simulink model "Mooventure2016_Rev5"  (Simulink 7.7)
settings: Solver=FixedStepDiscrete  StartTime=0.0  StopTime=10  RelTol=1e-3
PreLoadFcn:
  | try, eval([bdroot '_setup']); catch, eval('model_setup', ''); end
InitFcn:
  | try, eval([bdroot '_setup']); catch, eval('model_setup', ''); end
undefined symbols (not defined in the file): ECM, H1, motohawk_build_version, motohawk_trunc_name, motohawk_vardec_config_group, motohawk_vardec_path, xD
libraries: MotoHawk_lib x976, motohawk_control_primitives_lib x41, simulink x27, motohawk_annotations_lib x3
(part 14 of 16)

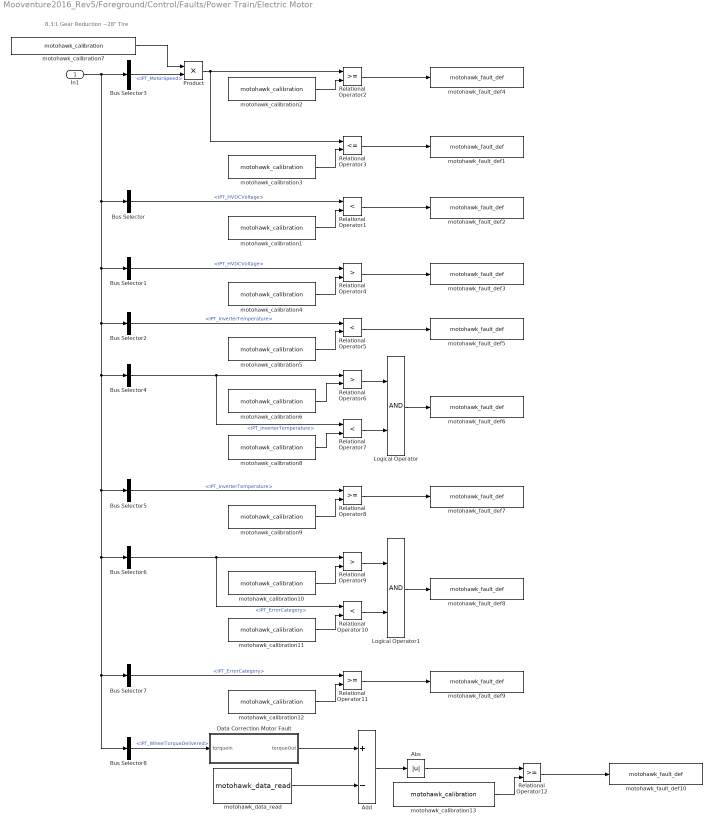
== system Mooventure2016_Rev5/Foreground/Control/Faults/Power Train/Electric Motor ==
  note: 8.3:1 Gear Reduction
      | ~28" Tire
  In1 : Inport
  Abs : Abs
  Add : Sum  Inputs=+-
  Bus Selector : BusSelector  OutputSignals=IPT.ID 278 IPT Status 1.IPT_HVDCVoltage
  Bus Selector1 : BusSelector  OutputSignals=IPT.ID 278 IPT Status 1.IPT_HVDCVoltage
  Bus Selector2 : BusSelector  OutputSignals=IPT.ID 278 IPT Status 1.IPT_InverterTemperature
  Bus Selector3 : BusSelector  OutputSignals=IPT.ID 260 IPT Status 2.IPT_MotorSpeed
  Bus Selector4 : BusSelector  OutputSignals=IPT.ID 278 IPT Status 1.IPT_InverterTemperature
  Bus Selector5 : BusSelector  OutputSignals=IPT.ID 278 IPT Status 1.IPT_InverterTemperature
  Bus Selector6 : BusSelector  OutputSignals=IPT.ID 278 IPT Status 1.IPT_ErrorCategory
  Bus Selector7 : BusSelector  OutputSignals=IPT.ID 278 IPT Status 1.IPT_ErrorCategory
  Bus Selector8 : BusSelector  OutputSignals=IPT.ID 260 IPT Status 2.IPT_WheelTorqueDelivered
  Data Correction Motor Fault : Stateflow chart  TreatAsAtomicUnit=on
  Logical Operator : Logic  AllPortsSameDT=off  OutDataTypeStr=boolean
  Logical Operator1 : Logic  AllPortsSameDT=off  OutDataTypeStr=boolean
  Product : Product  RndMeth=Zero
  Relational Operator{1,5,7,10} (4 alike) : RelationalOperator  Operator=<  OutDataTypeStr=boolean
  Relational Operator{2,8,11..12} (4 alike) : RelationalOperator  OutDataTypeStr=boolean
  Relational Operator3 : RelationalOperator  Operator=<=  OutDataTypeStr=boolean
  Relational Operator4 : RelationalOperator  Operator=>  OutDataTypeStr=boolean
  Relational Operator6 : RelationalOperator  Operator=>  OutDataTypeStr=boolean
  Relational Operator9 : RelationalOperator  Operator=>  OutDataTypeStr=boolean
  motohawk_calibration1 : MotoHawk_lib/Calibration & Probing Blocks/motohawk_calibration  nam='Electric_Motor_Derated_Under_Voltage_Fault'  val=250  storage=Calibration  show_more=off  name_source=Use Parameter  data_type=Inherit from 'Default Value'  read_level=1  write_level=1  ovr_cals=on  view_as=Number  enum_struct={'Disabled', 'Enabled'}  vector_style=Wide Row  use_help_units=off  help=''  units=''  use_header_enum=off  row_header_enum={}  col_header_enum={}  use_min_max=off  min_val=-inf  max_val=inf  use_precision=off  precision=''  gain=1  offset=0  exp=1  use_mototune_group=off  mototune_group=motohawk_vardec_path(gcb)
  motohawk_calibration10 : MotoHawk_lib/Calibration & Probing Blocks/motohawk_calibration  nam='Electric_Motor_General_Error_Fault_Under'  val=3  storage=Calibration  show_more=off  name_source=Use Parameter  data_type=Inherit from 'Default Value'  read_level=1  write_level=1  ovr_cals=on  view_as=Number  enum_struct={'Disabled', 'Enabled'}  vector_style=Wide Row  use_help_units=off  help=''  units=''  use_header_enum=off  row_header_enum={}  col_header_enum={}  use_min_max=off  min_val=-inf  max_val=inf  use_precision=off  precision=''  gain=1  offset=0  exp=1  use_mototune_group=off  mototune_group=motohawk_vardec_path(gcb)
  motohawk_calibration11 : MotoHawk_lib/Calibration & Probing Blocks/motohawk_calibration  nam='Electric_Motor_General_Error_Fault_Over'  val=8  storage=Calibration  show_more=off  name_source=Use Parameter  data_type=Inherit from 'Default Value'  read_level=1  write_level=1  ovr_cals=on  view_as=Number  enum_struct={'Disabled', 'Enabled'}  vector_style=Wide Row  use_help_units=off  help=''  units=''  use_header_enum=off  row_header_enum={}  col_header_enum={}  use_min_max=off  min_val=-inf  max_val=inf  use_precision=off  precision=''  gain=1  offset=0  exp=1  use_mototune_group=off  mototune_group=motohawk_vardec_path(gcb)
  motohawk_calibration12 : MotoHawk_lib/Calibration & Probing Blocks/motohawk_calibration  nam='Electric_Motor_Shutdown_Error_Fault'  val=8  storage=Calibration  show_more=off  name_source=Use Parameter  data_type=Inherit from 'Default Value'  read_level=1  write_level=1  ovr_cals=on  view_as=Number  enum_struct={'Disabled', 'Enabled'}  vector_style=Wide Row  use_help_units=off  help=''  units=''  use_header_enum=off  row_header_enum={}  col_header_enum={}  use_min_max=off  min_val=-inf  max_val=inf  use_precision=off  precision=''  gain=1  offset=0  exp=1  use_mototune_group=off  mototune_group=motohawk_vardec_path(gcb)
  motohawk_calibration13 : MotoHawk_lib/Calibration & Probing Blocks/motohawk_calibration  nam='Electric_Motor_Torque_Output_Fault'  val=200  storage=Calibration  show_more=off  name_source=Use Parameter  data_type=Inherit from 'Default Value'  read_level=1  write_level=1  ovr_cals=on  view_as=Number  enum_struct={'Disabled', 'Enabled'}  vector_style=Wide Row  use_help_units=off  help=''  units=''  use_header_enum=off  row_header_enum={}  col_header_enum={}  use_min_max=off  min_val=-inf  max_val=inf  use_precision=off  precision=''  gain=1  offset=0  exp=1  use_mototune_group=off  mototune_group=motohawk_vardec_path(gcb)
  motohawk_calibration2 : MotoHawk_lib/Calibration & Probing Blocks/motohawk_calibration  nam='Electric_Motor_Over_Speed_Forward_Fault'  val=120  storage=Calibration  show_more=off  name_source=Use Parameter  data_type=Inherit from 'Default Value'  read_level=1  write_level=1  ovr_cals=on  view_as=Number  enum_struct={'Disabled', 'Enabled'}  vector_style=Wide Row  use_help_units=off  help=''  units=''  use_header_enum=off  row_header_enum={}  col_header_enum={}  use_min_max=off  min_val=-inf  max_val=inf  use_precision=off  precision=''  gain=1  offset=0  exp=1  use_mototune_group=off  mototune_group=motohawk_vardec_path(gcb)
  motohawk_calibration3 : MotoHawk_lib/Calibration & Probing Blocks/motohawk_calibration  nam='Electric_Motor_Over_Speed_Reverse_Fault'  val=-40  storage=Calibration  show_more=off  name_source=Use Parameter  data_type=Inherit from 'Default Value'  read_level=1  write_level=1  ovr_cals=on  view_as=Number  enum_struct={'Disabled', 'Enabled'}  vector_style=Wide Row  use_help_units=off  help=''  units=''  use_header_enum=off  row_header_enum={}  col_header_enum={}  use_min_max=off  min_val=-inf  max_val=inf  use_precision=off  precision=''  gain=1  offset=0  exp=1  use_mototune_group=off  mototune_group=motohawk_vardec_path(gcb)
  motohawk_calibration4 : MotoHawk_lib/Calibration & Probing Blocks/motohawk_calibration  nam='Electric_Motor_Derated_Over_Voltage_Fault'  val=420  storage=Calibration  show_more=off  name_source=Use Parameter  data_type=Inherit from 'Default Value'  read_level=1  write_level=1  ovr_cals=on  view_as=Number  enum_struct={'Disabled', 'Enabled'}  vector_style=Wide Row  use_help_units=off  help=''  units=''  use_header_enum=off  row_header_enum={}  col_header_enum={}  use_min_max=off  min_val=-inf  max_val=inf  use_precision=off  precision=''  gain=1  offset=0  exp=1  use_mototune_group=off  mototune_group=motohawk_vardec_path(gcb)
  motohawk_calibration5 : MotoHawk_lib/Calibration & Probing Blocks/motohawk_calibration  nam='Electric_Motor_Derated_Under_Temperature_Fault'  val=-25  storage=Calibration  show_more=off  name_source=Use Parameter  data_type=Inherit from 'Default Value'  read_level=1  write_level=1  ovr_cals=on  view_as=Number  enum_struct={'Disabled', 'Enabled'}  vector_style=Wide Row  use_help_units=off  help=''  units=''  use_header_enum=off  row_header_enum={}  col_header_enum={}  use_min_max=off  min_val=-inf  max_val=inf  use_precision=off  precision=''  gain=1  offset=0  exp=1  use_mototune_group=off  mototune_group=motohawk_vardec_path(gcb)
  motohawk_calibration6 : MotoHawk_lib/Calibration & Probing Blocks/motohawk_calibration  nam='Electric_Motor_Derated_Approaching_Over_Temperature_Fault_Under'  val=50  storage=Calibration  show_more=off  name_source=Use Parameter  data_type=Inherit from 'Default Value'  read_level=1  write_level=1  ovr_cals=on  view_as=Number  enum_struct={'Disabled', 'Enabled'}  vector_style=Wide Row  use_help_units=off  help=''  units=''  use_header_enum=off  row_header_enum={}  col_header_enum={}  use_min_max=off  min_val=-inf  max_val=inf  use_precision=off  precision=''  gain=1  offset=0  exp=1  use_mototune_group=off  mototune_group=motohawk_vardec_path(gcb)
  motohawk_calibration7 : MotoHawk_lib/Calibration & Probing Blocks/motohawk_calibration  nam='RPM_to_Wheel_Speed_Multiplier2'  val=0.01001896  storage=Calibration  show_more=off  name_source=Use Parameter  data_type=Inherit from 'Default Value'  read_level=1  write_level=1  ovr_cals=on  view_as=Number  enum_struct={'Disabled', 'Enabled'}  vector_style=Wide Row  use_help_units=off  help=''  units=''  use_header_enum=off  row_header_enum={}  col_header_enum={}  use_min_max=off  min_val=-inf  max_val=inf  use_precision=off  precision=''  gain=1  offset=0  exp=1  use_mototune_group=off  mototune_group=motohawk_vardec_path(gcb)
  motohawk_calibration8 : MotoHawk_lib/Calibration & Probing Blocks/motohawk_calibration  nam='Electric_Motor_Derated_Approaching_Over_Temperature_Fault_Over'  val=65  storage=Calibration  show_more=off  name_source=Use Parameter  data_type=Inherit from 'Default Value'  read_level=1  write_level=1  ovr_cals=on  view_as=Number  enum_struct={'Disabled', 'Enabled'}  vector_style=Wide Row  use_help_units=off  help=''  units=''  use_header_enum=off  row_header_enum={}  col_header_enum={}  use_min_max=off  min_val=-inf  max_val=inf  use_precision=off  precision=''  gain=1  offset=0  exp=1  use_mototune_group=off  mototune_group=motohawk_vardec_path(gcb)
  motohawk_calibration9 : MotoHawk_lib/Calibration & Probing Blocks/motohawk_calibration  nam='Electric_Motor_Derated_Over_Temperature_Fault'  val=65  storage=Calibration  show_more=off  name_source=Use Parameter  data_type=Inherit from 'Default Value'  read_level=1  write_level=1  ovr_cals=on  view_as=Number  enum_struct={'Disabled', 'Enabled'}  vector_style=Wide Row  use_help_units=off  help=''  units=''  use_header_enum=off  row_header_enum={}  col_header_enum={}  use_min_max=off  min_val=-inf  max_val=inf  use_precision=off  precision=''  gain=1  offset=0  exp=1  use_mototune_group=off  mototune_group=motohawk_vardec_path(gcb)
  motohawk_data_read : MotoHawk_lib/Data Storage Blocks/motohawk_data_read  source=Lookup By Name  structure=Scalar  operation=Read scalar from location by index  sz_vec=4  sz_row=2  sz_col=3  typ=double  nam='TorqueRequest'  checkNull=on  struct_inst_name='MyData'  struct_nam='MyStruct'
  motohawk_fault_def1 : MotoHawk_lib/Fault Management Blocks/motohawk_fault_def  nam='Electric_Motor_Over_Speed_Reverse'  mode=Enabled  id=['P1A11']  x=5  y=10  input_suspected=on  indeterminate=off  increment_xy=on  downsample_count=1  ovr_cals=on  ovr_actions=on  show_actions=on  action1_name='Wrench_Light'  action1_cond=Active  action2_name=''  action2_cond=(None)  action3_name=''  action3_cond=(None)  action4_name=''  action4_cond=(None)
  motohawk_fault_def10 : MotoHawk_lib/Fault Management Blocks/motohawk_fault_def  nam='Electric_Motor_Torque_Output_Fault'  mode=Disabled  id=['P1A50']  x=900  y=2500  input_suspected=on  indeterminate=off  increment_xy=on  downsample_count=1  ovr_cals=on  ovr_actions=on  show_actions=on  action1_name='Wrench_Light'  action1_cond=Active  action2_name=''  action2_cond=(None)  action3_name=''  action3_cond=(None)  action4_name=''  action4_cond=(None)
  motohawk_fault_def2 : MotoHawk_lib/Fault Management Blocks/motohawk_fault_def  nam='Electric_Motor_Derated_Under_Voltage'  mode=Enabled  id=['P1A20']  x=500  y=1000  input_suspected=on  indeterminate=off  increment_xy=on  downsample_count=1  ovr_cals=on  ovr_actions=on  show_actions=on  action1_name='Check_Engine_Light_Flashing'  action1_cond=Active  action2_name=''  action2_cond=(None)  action3_name=''  action3_cond=(None)  action4_name=''  action4_cond=(None)
  motohawk_fault_def3 : MotoHawk_lib/Fault Management Blocks/motohawk_fault_def  nam='Electric_Motor_Derated_Over_Voltage'  mode=Enabled  id=['P1A21']  x=500  y=1000  input_suspected=on  indeterminate=off  increment_xy=on  downsample_count=1  ovr_cals=on  ovr_actions=on  show_actions=on  action1_name='Check_Engine_Light'  action1_cond=Active  action2_name='Dyno_Shutdown'  action2_cond=Active  action3_name=''  action3_cond=(None)  action4_name=''  action4_cond=(None)
  motohawk_fault_def4 : MotoHawk_lib/Fault Management Blocks/motohawk_fault_def  nam='Electric_Motor_Over_Speed_Forward'  mode=Enabled  id=['P1A10']  x=5  y=10  input_suspected=on  indeterminate=off  increment_xy=on  downsample_count=1  ovr_cals=on  ovr_actions=on  show_actions=on  action1_name='Wrench_Light'  action1_cond=Active  action2_name=''  action2_cond=(None)  action3_name=''  action3_cond=(None)  action4_name=''  action4_cond=(None)
  motohawk_fault_def5 : MotoHawk_lib/Fault Management Blocks/motohawk_fault_def  nam='Electric_Motor_Derated_Under_Temperature'  mode=Enabled  id=['P1A22']  x=9  y=10  input_suspected=on  indeterminate=off  increment_xy=on  downsample_count=1  ovr_cals=on  ovr_actions=on  show_actions=on  action1_name='Temperature_Flash'  action1_cond=Active  action2_name=''  action2_cond=(None)  action3_name=''  action3_cond=(None)  action4_name=''  action4_cond=(None)
  motohawk_fault_def6 : MotoHawk_lib/Fault Management Blocks/motohawk_fault_def  nam='Electric_Motor_Approaching_Over_Temperature'  mode=Enabled  id=['P1A22']  x=9  y=10  input_suspected=on  indeterminate=off  increment_xy=on  downsample_count=1  ovr_cals=on  ovr_actions=on  show_actions=on  action1_name='Temperature_Flash'  action1_cond=Active  action2_name='Cooling_Max'  action2_cond=Active  action3_name=''  action3_cond=(None)  action4_name=''  action4_cond=(None)
  motohawk_fault_def7 : MotoHawk_lib/Fault Management Blocks/motohawk_fault_def  nam='Electric_Motor_Derated_Over_Temperature'  mode=Enabled  id=['P1A24']  x=9  y=10  input_suspected=on  indeterminate=off  increment_xy=on  downsample_count=1  ovr_cals=on  ovr_actions=on  show_actions=on  action1_name='Temperature_Solid'  action1_cond=Active  action2_name='Dyno_Shutdown'  action2_cond=Active  action3_name='Cooling_Max'  action3_cond=Active  action4_name=''  action4_cond=(None)
  motohawk_fault_def8 : MotoHawk_lib/Fault Management Blocks/motohawk_fault_def  nam='Electric_Motor_General_Error'  mode=Enabled  id=['P1A30']  x=9  y=10  input_suspected=on  indeterminate=off  increment_xy=on  downsample_count=1  ovr_cals=on  ovr_actions=on  show_actions=on  action1_name='Check_Engine_Light'  action1_cond=Active  action2_name=''  action2_cond=(None)  action3_name=''  action3_cond=(None)  action4_name=''  action4_cond=(None)
  motohawk_fault_def9 : MotoHawk_lib/Fault Management Blocks/motohawk_fault_def  nam='Electric_Motor_Shutodwn_Error'  mode=Enabled  id=['P1A31']  x=9  y=10  input_suspected=on  indeterminate=off  increment_xy=on  downsample_count=1  ovr_cals=on  ovr_actions=on  show_actions=on  action1_name='Check_Engine_Light_Flashing'  action1_cond=Active  action2_name=''  action2_cond=(None)  action3_name=''  action3_cond=(None)  action4_name=''  action4_cond=(None)
  wires:
  Bus Selector3/1 -> Product/2  "<IPT_MotorSpeed>"
  motohawk_calibration7/1 -> Product/1
  In1/1 -> Bus Selector3/1, Bus Selector/1, Bus Selector1/1, Bus Selector2/1, Bus Selector4/1, Bus Selector5/1, Bus Selector6/1, Bus Selector7/1, Bus Selector8/1
  motohawk_calibration2/1 -> Relational Operator2/2
  Relational Operator2/1 -> motohawk_fault_def4/1
  motohawk_calibration3/1 -> Relational Operator3/2
  Relational Operator3/1 -> motohawk_fault_def1/1
  Product/1 -> Relational Operator2/1, Relational Operator3/1
  motohawk_calibration1/1 -> Relational Operator1/2
  Relational Operator1/1 -> motohawk_fault_def2/1
  Bus Selector/1 -> Relational Operator1/1  "<IPT_HVDCVoltage>"
  motohawk_calibration4/1 -> Relational Operator4/2
  Relational Operator4/1 -> motohawk_fault_def3/1
  Bus Selector1/1 -> Relational Operator4/1  "<IPT_HVDCVoltage>"
  motohawk_calibration5/1 -> Relational Operator5/2
  Relational Operator5/1 -> motohawk_fault_def5/1
  Bus Selector2/1 -> Relational Operator5/1  "<IPT_InverterTemperature>"
  motohawk_calibration6/1 -> Relational Operator6/2
  Bus Selector4/1 -> Relational Operator6/1, Relational Operator7/1  "<IPT_InverterTemperature>"
  motohawk_calibration8/1 -> Relational Operator7/2
  Relational Operator7/1 -> Logical Operator/2
  Relational Operator6/1 -> Logical Operator/1
  Logical Operator/1 -> motohawk_fault_def6/1
  motohawk_calibration9/1 -> Relational Operator8/2
  Relational Operator8/1 -> motohawk_fault_def7/1
  Bus Selector5/1 -> Relational Operator8/1  "<IPT_InverterTemperature>"
  motohawk_calibration10/1 -> Relational Operator9/2
  Bus Selector6/1 -> Relational Operator9/1, Relational Operator10/1  "<IPT_ErrorCategory>"
  motohawk_calibration11/1 -> Relational Operator10/2
  Relational Operator10/1 -> Logical Operator1/2
  Relational Operator9/1 -> Logical Operator1/1
  Logical Operator1/1 -> motohawk_fault_def8/1
  motohawk_calibration12/1 -> Relational Operator11/2
  Relational Operator11/1 -> motohawk_fault_def9/1
  Bus Selector7/1 -> Relational Operator11/1  "<IPT_ErrorCategory>"
  Add/1 -> Abs/1
  motohawk_calibration13/1 -> Relational Operator12/2
  Abs/1 -> Relational Operator12/1
  Relational Operator12/1 -> motohawk_fault_def10/1
  motohawk_data_read/1 -> Add/2
  Bus Selector8/1 -> Data Correction Motor Fault/1(torqueIn)  "<IPT_WheelTorqueDelivered>"
  Data Correction Motor Fault/1(torqueOut) -> Add/1

== system Mooventure2016_Rev5/Foreground/Control/Faults/Power Train/Gas Pedal ==
  In1 : Inport
  Abs : Abs
  Add : Sum  Inputs=+-
  Bus Selector : BusSelector  OutputSignals=Driver Inputs.Throttle_Position (signal 5)
  Bus Selector2 : BusSelector  OutputSignals=Driver Inputs.Throttle_Position (signal 5)
  Bus Selector3 : BusSelector  OutputSignals=Driver Inputs.Throttle_Position (signal 5)
  Relational Operator : RelationalOperator  OutDataTypeStr=boolean
  Relational Operator2 : RelationalOperator  Operator=<=  OutDataTypeStr=boolean
  Relational Operator3 : RelationalOperator  OutDataTypeStr=boolean
  Unit Delay : UnitDelay  SampleTime=-1
  motohawk_calibration : MotoHawk_lib/Calibration & Probing Blocks/motohawk_calibration  nam='Pedal_Poition_Sensor_A_Intermittent'  val=15  storage=Calibration  show_more=off  name_source=Use Parameter  data_type=Inherit from 'Default Value'  read_level=1  write_level=1  ovr_cals=on  view_as=Number  enum_struct={'Disabled', 'Enabled'}  vector_style=Wide Row  use_help_units=off  help=''  units=''  use_header_enum=off  row_header_enum={}  col_header_enum={}  use_min_max=off  min_val=-inf  max_val=inf  use_precision=off  precision=''  gain=1  offset=0  exp=1  use_mototune_group=off  mototune_group=motohawk_vardec_path(gcb)
  motohawk_calibration2 : MotoHawk_lib/Calibration & Probing Blocks/motohawk_calibration  nam='Pedal_Position_Sensor_A_Circuit_Low'  val=0  storage=Calibration  show_more=off  name_source=Use Parameter  data_type=Inherit from 'Default Value'  read_level=1  write_level=1  ovr_cals=on  view_as=Number  enum_struct={'Disabled', 'Enabled'}  vector_style=Wide Row  use_help_units=off  help=''  units=''  use_header_enum=off  row_header_enum={}  col_header_enum={}  use_min_max=off  min_val=-inf  max_val=inf  use_precision=off  precision=''  gain=1  offset=0  exp=1  use_mototune_group=off  mototune_group=motohawk_vardec_path(gcb)
  motohawk_calibration3 : MotoHawk_lib/Calibration & Probing Blocks/motohawk_calibration  nam='Pedal_Position_Sensor_A_Circuit_High'  val=130  storage=Calibration  show_more=off  name_source=Use Parameter  data_type=Inherit from 'Default Value'  read_level=1  write_level=1  ovr_cals=on  view_as=Number  enum_struct={'Disabled', 'Enabled'}  vector_style=Wide Row  use_help_units=off  help=''  units=''  use_header_enum=off  row_header_enum={}  col_header_enum={}  use_min_max=off  min_val=-inf  max_val=inf  use_precision=off  precision=''  gain=1  offset=0  exp=1  use_mototune_group=off  mototune_group=motohawk_vardec_path(gcb)
  motohawk_fault_def1 : MotoHawk_lib/Fault Management Blocks/motohawk_fault_def  nam='Pedal_Position_Sensor_A_Circuit_High'  mode=Enabled  id=['P1512']  x=5  y=10  input_suspected=on  indeterminate=off  increment_xy=on  downsample_count=1  ovr_cals=on  ovr_actions=on  show_actions=on  action1_name='Wrench_Light'  action1_cond=Active  action2_name='Dyno_Shutdown'  action2_cond=(None)  action3_name=''  action3_cond=(None)  action4_name=''  action4_cond=(None)
  motohawk_fault_def2 : MotoHawk_lib/Fault Management Blocks/motohawk_fault_def  nam='Pedal_Position_Sensor_A_Circuit_Intermittent'  mode=Disabled  id=['P1510']  x=90  y=250  input_suspected=on  indeterminate=off  increment_xy=on  downsample_count=4  ovr_cals=on  ovr_actions=on  show_actions=on  action1_name='Wrench_Light'  action1_cond=Active  action2_name=''  action2_cond=(None)  action3_name=''  action3_cond=(None)  action4_name=''  action4_cond=(None)
  motohawk_fault_def4 : MotoHawk_lib/Fault Management Blocks/motohawk_fault_def  nam='Pedal_Position_Sensor_A_Circuit_Low'  mode=Enabled  id=['P1511']  x=5  y=10  input_suspected=on  indeterminate=off  increment_xy=on  downsample_count=1  ovr_cals=on  ovr_actions=on  show_actions=on  action1_name='Wrench_Light'  action1_cond=Active  action2_name=''  action2_cond=(None)  action3_name=''  action3_cond=(None)  action4_name=''  action4_cond=(None)
  wires:
  In1/1 -> Bus Selector/1, Bus Selector2/1, Bus Selector3/1
  Bus Selector/1 -> Add/1, Unit Delay/1  "<Throttle_Position (signal 5)>"
  Unit Delay/1 -> Add/2
  Add/1 -> Abs/1
  Abs/1 -> Relational Operator/1
  Relational Operator/1 -> motohawk_fault_def2/1
  motohawk_calibration/1 -> Relational Operator/2
  motohawk_calibration2/1 -> Relational Operator2/2
  Relational Operator2/1 -> motohawk_fault_def4/1
  Bus Selector3/1 -> Relational Operator3/1  "<Throttle_Position (signal 5)>"
  motohawk_calibration3/1 -> Relational Operator3/2
  Relational Operator3/1 -> motohawk_fault_def1/1
  Bus Selector2/1 -> Relational Operator2/1  "<Throttle_Position (signal 5)>"

== system Mooventure2016_Rev5/Foreground/Control/Faults/Power Train/Gear Selector ==
  In1 : Inport
  Bus Selector{,1..3} (4 alike) : BusSelector  OutputSignals=Driver Inputs.Shift_Position (signal 4)
  Bus Selector4 : BusSelector  OutputSignals=Driver Inputs.AgeCount (signal 3)
  Logical Operator1 : Logic  Operator=OR  AllPortsSameDT=off  OutDataTypeStr=boolean
  Logical Operator2 : Logic  Operator=OR  AllPortsSameDT=off  OutDataTypeStr=boolean
  Relational Operator : RelationalOperator  Operator=<=  OutDataTypeStr=boolean
  Relational Operator1 : RelationalOperator  OutDataTypeStr=boolean
  Relational Operator2 : RelationalOperator  Operator=<=  OutDataTypeStr=boolean
  Relational Operator3 : RelationalOperator  OutDataTypeStr=boolean
  Relational Operator4 : RelationalOperator  OutDataTypeStr=boolean
  motohawk_calibration : MotoHawk_lib/Calibration & Probing Blocks/motohawk_calibration  nam='Park_Nuetral_Switch_Input_Low_Fault'  val=0  storage=Calibration  show_more=off  name_source=Use Parameter  data_type=Inherit from 'Default Value'  read_level=1  write_level=1  ovr_cals=on  view_as=Number  enum_struct={'Disabled', 'Enabled'}  vector_style=Wide Row  use_help_units=off  help=''  units=''  use_header_enum=off  row_header_enum={}  col_header_enum={}  use_min_max=off  min_val=-inf  max_val=inf  use_precision=off  precision=''  gain=1  offset=0  exp=1  use_mototune_group=off  mototune_group=motohawk_vardec_path(gcb)
  motohawk_calibration1 : MotoHawk_lib/Calibration & Probing Blocks/motohawk_calibration  nam='Park_Nuetral_Switch_Input_High_Fault'  val=13  storage=Calibration  show_more=off  name_source=Use Parameter  data_type=Inherit from 'Default Value'  read_level=1  write_level=1  ovr_cals=on  view_as=Number  enum_struct={'Disabled', 'Enabled'}  vector_style=Wide Row  use_help_units=off  help=''  units=''  use_header_enum=off  row_header_enum={}  col_header_enum={}  use_min_max=off  min_val=-inf  max_val=inf  use_precision=off  precision=''  gain=1  offset=0  exp=1  use_mototune_group=off  mototune_group=motohawk_vardec_path(gcb)
  motohawk_calibration2 : MotoHawk_lib/Calibration & Probing Blocks/motohawk_calibration  nam='Drive_Switch_Input_Low_Fault'  val=0  storage=Calibration  show_more=off  name_source=Use Parameter  data_type=Inherit from 'Default Value'  read_level=1  write_level=1  ovr_cals=on  view_as=Number  enum_struct={'Disabled', 'Enabled'}  vector_style=Wide Row  use_help_units=off  help=''  units=''  use_header_enum=off  row_header_enum={}  col_header_enum={}  use_min_max=off  min_val=-inf  max_val=inf  use_precision=off  precision=''  gain=1  offset=0  exp=1  use_mototune_group=off  mototune_group=motohawk_vardec_path(gcb)
  motohawk_calibration3 : MotoHawk_lib/Calibration & Probing Blocks/motohawk_calibration  nam='Drive_Switch_Input_High_Fault'  val=13  storage=Calibration  show_more=off  name_source=Use Parameter  data_type=Inherit from 'Default Value'  read_level=1  write_level=1  ovr_cals=on  view_as=Number  enum_struct={'Disabled', 'Enabled'}  vector_style=Wide Row  use_help_units=off  help=''  units=''  use_header_enum=off  row_header_enum={}  col_header_enum={}  use_min_max=off  min_val=-inf  max_val=inf  use_precision=off  precision=''  gain=1  offset=0  exp=1  use_mototune_group=off  mototune_group=motohawk_vardec_path(gcb)
  motohawk_calibration4 : MotoHawk_lib/Calibration & Probing Blocks/motohawk_calibration  nam='Gear_Shift_Module_Communication_Circuit'  val=1000  storage=Calibration  show_more=off  name_source=Use Parameter  data_type=Inherit from 'Default Value'  read_level=1  write_level=1  ovr_cals=on  view_as=Number  enum_struct={'Disabled', 'Enabled'}  vector_style=Wide Row  use_help_units=off  help=''  units=''  use_header_enum=off  row_header_enum={}  col_header_enum={}  use_min_max=off  min_val=-inf  max_val=inf  use_precision=off  precision=''  gain=1  offset=0  exp=1  use_mototune_group=off  mototune_group=motohawk_vardec_path(gcb)
  motohawk_fault_def1 : MotoHawk_lib/Fault Management Blocks/motohawk_fault_def  nam='Park_Nuetral_Switch_Input_High'  mode=Enabled  id=['P0852']  x=5  y=10  input_suspected=on  indeterminate=off  increment_xy=on  downsample_count=1  ovr_cals=on  ovr_actions=on  show_actions=on  action1_name='Wrench_Light'  action1_cond=Active  action2_name=''  action2_cond=(None)  action3_name=''  action3_cond=(None)  action4_name=''  action4_cond=(None)
  motohawk_fault_def2 : MotoHawk_lib/Fault Management Blocks/motohawk_fault_def  nam='Drive_Switch_Input_High'  mode=Enabled  id=['P0855']  x=5  y=10  input_suspected=on  indeterminate=off  increment_xy=on  downsample_count=1  ovr_cals=on  ovr_actions=on  show_actions=on  action1_name='Wrench_Light'  action1_cond=Active  action2_name=''  action2_cond=(None)  action3_name=''  action3_cond=(None)  action4_name=''  action4_cond=(None)
  motohawk_fault_def3 : MotoHawk_lib/Fault Management Blocks/motohawk_fault_def  nam='Drive_Switch_Input_Circuit'  mode=Enabled  id=['P0853']  x=9  y=10  input_suspected=on  indeterminate=off  increment_xy=on  downsample_count=1  ovr_cals=on  ovr_actions=on  show_actions=on  action1_name=''  action1_cond=(None)  action2_name=''  action2_cond=(None)  action3_name=''  action3_cond=(None)  action4_name=''  action4_cond=(None)
  motohawk_fault_def4 : MotoHawk_lib/Fault Management Blocks/motohawk_fault_def  nam='Drive_Switch_Input_Low'  mode=Enabled  id=['P0854']  x=5  y=10  input_suspected=on  indeterminate=off  increment_xy=on  downsample_count=1  ovr_cals=on  ovr_actions=on  show_actions=on  action1_name='Wrench_Light'  action1_cond=Active  action2_name=''  action2_cond=(None)  action3_name=''  action3_cond=(None)  action4_name=''  action4_cond=(None)
  motohawk_fault_def5 : MotoHawk_lib/Fault Management Blocks/motohawk_fault_def  nam='Gear_Shift_Communication_Circuit'  mode=Enabled  id=['P0860']  x=5  y=10  input_suspected=on  indeterminate=off  increment_xy=on  downsample_count=1  ovr_cals=on  ovr_actions=on  show_actions=on  action1_name='Wrench_Light'  action1_cond=Active  action2_name=''  action2_cond=(None)  action3_name=''  action3_cond=(None)  action4_name=''  action4_cond=(None)
  motohawk_fault_def7 : MotoHawk_lib/Fault Management Blocks/motohawk_fault_def  nam='Park_Nuetral_Switch_Input_Circuit'  mode=Enabled  id=['P0850']  x=9  y=10  input_suspected=on  indeterminate=off  increment_xy=on  downsample_count=1  ovr_cals=on  ovr_actions=on  show_actions=on  action1_name=''  action1_cond=(None)  action2_name=''  action2_cond=(None)  action3_name=''  action3_cond=(None)  action4_name=''  action4_cond=(None)
  motohawk_fault_def8 : MotoHawk_lib/Fault Management Blocks/motohawk_fault_def  nam='Park_Nuetral_Switch_Input_Low'  mode=Enabled  id=['P0851']  x=5  y=10  input_suspected=on  indeterminate=off  increment_xy=on  downsample_count=1  ovr_cals=on  ovr_actions=on  show_actions=on  action1_name='Wrench_Light'  action1_cond=Active  action2_name=''  action2_cond=(None)  action3_name=''  action3_cond=(None)  action4_name=''  action4_cond=(None)
  wires:
  In1/1 -> Bus Selector/1, Bus Selector1/1, Bus Selector2/1, Bus Selector3/1, Bus Selector4/1
  Bus Selector/1 -> Relational Operator/1  "<Shift_Position (signal 4)>"
  motohawk_calibration/1 -> Relational Operator/2
  Relational Operator/1 -> motohawk_fault_def8/1, Logical Operator2/2
  Bus Selector1/1 -> Relational Operator1/1  "<Shift_Position (signal 4)>"
  motohawk_calibration1/1 -> Relational Operator1/2
  Relational Operator1/1 -> motohawk_fault_def1/1, Logical Operator2/1
  Logical Operator2/1 -> motohawk_fault_def7/1
  Bus Selector2/1 -> Relational Operator2/1  "<Shift_Position (signal 4)>"
  motohawk_calibration2/1 -> Relational Operator2/2
  Relational Operator2/1 -> motohawk_fault_def4/1, Logical Operator1/1, Logical Operator1/2
  Bus Selector3/1 -> Relational Operator3/1  "<Shift_Position (signal 4)>"
  motohawk_calibration3/1 -> Relational Operator3/2
  Relational Operator3/1 -> motohawk_fault_def2/1
  Logical Operator1/1 -> motohawk_fault_def3/1
  Bus Selector4/1 -> Relational Operator4/1  "<AgeCount (signal 3)>"
  motohawk_calibration4/1 -> Relational Operator4/2
  Relational Operator4/1 -> motohawk_fault_def5/1

== system Mooventure2016_Rev5/Foreground/Control/Faults/Power Train/Ignition Key ==
  Logical Operator : Logic  AllPortsSameDT=off  OutDataTypeStr=boolean
  Relational Operator1 : RelationalOperator  OutDataTypeStr=boolean
  Relational Operator2 : RelationalOperator  OutDataTypeStr=boolean
  motohawk_calibration1 : MotoHawk_lib/Calibration & Probing Blocks/motohawk_calibration  nam='Key_Line_Voltage_Fault'  val=900  storage=Calibration  show_more=off  name_source=Use Parameter  data_type=Inherit from 'Default Value'  read_level=1  write_level=1  ovr_cals=on  view_as=Number  enum_struct={'Disabled', 'Enabled'}  vector_style=Wide Row  use_help_units=off  help=''  units=''  use_header_enum=off  row_header_enum={}  col_header_enum={}  use_min_max=off  min_val=-inf  max_val=inf  use_precision=off  precision=''  gain=1  offset=0  exp=1  use_mototune_group=off  mototune_group=motohawk_vardec_path(gcb)
  motohawk_calibration2 : MotoHawk_lib/Calibration & Probing Blocks/motohawk_calibration  nam='Key_Off_Coltage_High_Fault'  val=100  storage=Calibration  show_more=off  name_source=Use Parameter  data_type=Inherit from 'Default Value'  read_level=1  write_level=1  ovr_cals=on  view_as=Number  enum_struct={'Disabled', 'Enabled'}  vector_style=Wide Row  use_help_units=off  help=''  units=''  use_header_enum=off  row_header_enum={}  col_header_enum={}  use_min_max=off  min_val=-inf  max_val=inf  use_precision=off  precision=''  gain=1  offset=0  exp=1  use_mototune_group=off  mototune_group=motohawk_vardec_path(gcb)
  motohawk_data_read : MotoHawk_lib/Data Storage Blocks/motohawk_data_read  source=Lookup By Name  structure=Scalar  operation=Read scalar from location by index  sz_vec=4  sz_row=2  sz_col=3  typ=boolean  nam='Shutdown_Req'  checkNull=on  struct_inst_name='MyData'  struct_nam='MyStruct'
  motohawk_data_read1 : MotoHawk_lib/Data Storage Blocks/motohawk_data_read  source=Lookup By Name  structure=Scalar  operation=Read scalar from location by index  sz_vec=4  sz_row=2  sz_col=3  typ=double  nam='ECUP'  checkNull=on  struct_inst_name='MyData'  struct_nam='MyStruct'
  motohawk_fault_def1 : MotoHawk_lib/Fault Management Blocks/motohawk_fault_def  nam='Key_Line_Voltage'  mode=Enabled  id=['P1310']  x=5  y=10  input_suspected=on  indeterminate=off  increment_xy=on  downsample_count=1  ovr_cals=on  ovr_actions=on  show_actions=on  action1_name='Wrench_Light'  action1_cond=Active  action2_name=''  action2_cond=(None)  action3_name=''  action3_cond=(None)  action4_name=''  action4_cond=(None)
  motohawk_fault_def2 : MotoHawk_lib/Fault Management Blocks/motohawk_fault_def  nam='Key_Off_Voltage_High'  mode=Sticky  id=['P1311']  x=5  y=10  input_suspected=on  indeterminate=off  increment_xy=on  downsample_count=1  ovr_cals=on  ovr_actions=on  show_actions=on  action1_name=''  action1_cond=(None)  action2_name=''  action2_cond=(None)  action3_name=''  action3_cond=(None)  action4_name=''  action4_cond=(None)
  wires:
  motohawk_calibration1/1 -> Relational Operator1/2
  Relational Operator1/1 -> motohawk_fault_def1/1
  motohawk_calibration2/1 -> Relational Operator2/2
  Relational Operator2/1 -> Logical Operator/1
  motohawk_data_read/1 -> Logical Operator/2
  Logical Operator/1 -> motohawk_fault_def2/1
  motohawk_data_read1/1 -> Relational Operator1/1, Relational Operator2/1

== system Mooventure2016_Rev5/Foreground/Control/Faults/Power Train/Traction Control ==
  In1 : Inport
  Abs{,1..3} (4 alike) : Abs
  Bus Selector : BusSelector  OutputSignals=ABS.Wheel Speed.Front left whl speed,ABS.Wheel Speed.Front right whl speed,ABS.Wheel Speed.Rear left whl speed,ABS.Wheel Speed.Rear right whl speed
  Derivitive{,1..3} (4 alike) : motohawk_control_primitives_lib/Derivitive  SystemSampleTime=-1  samp_time=-1
  Logical Operator : Logic  Operator=OR  Inputs=4  AllPortsSameDT=off  OutDataTypeStr=boolean
  Relational Operator{,1..3} (4 alike) : RelationalOperator  Operator=>  OutDataTypeStr=boolean
  motohawk_calibration : MotoHawk_lib/Calibration & Probing Blocks/motohawk_calibration  nam='Traction_Control_System_Maulfunction_Fault'  val=35.28  storage=Calibration  show_more=off  name_source=Use Parameter  data_type=Inherit from 'Default Value'  read_level=1  write_level=1  ovr_cals=on  view_as=Number  enum_struct={'Disabled', 'Enabled'}  vector_style=Wide Row  use_help_units=off  help=''  units=''  use_header_enum=off  row_header_enum={}  col_header_enum={}  use_min_max=off  min_val=-inf  max_val=inf  use_precision=off  precision=''  gain=1  offset=0  exp=1  use_mototune_group=off  mototune_group=motohawk_vardec_path(gcb)
  motohawk_fault_def1 : MotoHawk_lib/Fault Management Blocks/motohawk_fault_def  nam='Traction_Control_Malfunction'  mode=Disabled  id=['P1520']  x=1000  y=2000  input_suspected=on  indeterminate=off  increment_xy=on  downsample_count=1  ovr_cals=on  ovr_actions=on  show_actions=on  action1_name='Wrench_Light'  action1_cond=Active  action2_name=''  action2_cond=(None)  action3_name=''  action3_cond=(None)  action4_name=''  action4_cond=(None)
  wires:
  In1/1 -> Bus Selector/1
  Bus Selector/1 -> Abs/1  "<Front left whl speed>"
  Abs/1 -> Derivitive/1
  Abs1/1 -> Derivitive1/1
  Abs2/1 -> Derivitive2/1
  Abs3/1 -> Derivitive3/1
  Bus Selector/4 -> Abs3/1  "<Rear right whl speed>"
  Bus Selector/3 -> Abs2/1  "<Rear left whl speed>"
  Bus Selector/2 -> Abs1/1  "<Front right whl speed>"
  Derivitive/1 -> Relational Operator/1
  Derivitive1/1 -> Relational Operator1/1
  Derivitive2/1 -> Relational Operator2/1
  Derivitive3/1 -> Relational Operator3/1
  motohawk_calibration/1 -> Relational Operator/2, Relational Operator1/2, Relational Operator2/2, Relational Operator3/2
  Relational Operator/1 -> Logical Operator/1
  Relational Operator1/1 -> Logical Operator/2
  Relational Operator2/1 -> Logical Operator/3
  Relational Operator3/1 -> Logical Operator/4
  Logical Operator/1 -> motohawk_fault_def1/1

== system Mooventure2016_Rev5/Foreground/Control/Faults/Power Train/Vehicle Speed Sensor ==
  In1 : Inport
  Abs : Abs
  Add : Sum  Inputs=+-
  Bus Selector1 : BusSelector  OutputSignals=IPT.ID 260 IPT Status 2.IPT_WheelTorqueDelivered,IPT.ID 260 IPT Status 2.IPT_MotorSpeed
  Bus Selector2 : BusSelector  OutputSignals=IPT.ID 260 IPT Status 2.IPT_MotorSpeed
  Bus Selector4 : BusSelector  OutputSignals=IPT.ID 260 IPT Status 2.IPT_MotorSpeed
  Data Correction : Stateflow chart  TreatAsAtomicUnit=on
  Logical Operator : Logic  Operator=OR  AllPortsSameDT=off  OutDataTypeStr=boolean
  Logical Operator1 : Logic  AllPortsSameDT=off  OutDataTypeStr=boolean
  Logical Operator2 : Logic  Operator=OR  Inputs=3  AllPortsSameDT=off  OutDataTypeStr=boolean
  Relational Operator : RelationalOperator  OutDataTypeStr=boolean
  Relational Operator1 : RelationalOperator  Operator=>  OutDataTypeStr=boolean
  Relational Operator2 : RelationalOperator  Operator=>  OutDataTypeStr=boolean
  Relational Operator3 : RelationalOperator  Operator=<  OutDataTypeStr=boolean
  Relational Operator7 : RelationalOperator  Operator=<  OutDataTypeStr=boolean
  Unit Delay : UnitDelay  SampleTime=-1
  motohawk_calibration1 : MotoHawk_lib/Calibration & Probing Blocks/motohawk_calibration  nam='Motor_Speed_High_Fault'  val=12500  storage=Calibration  show_more=off  name_source=Use Parameter  data_type=Inherit from 'Default Value'  read_level=1  write_level=1  ovr_cals=on  view_as=Number  enum_struct={'Disabled', 'Enabled'}  vector_style=Wide Row  use_help_units=off  help=''  units=''  use_header_enum=off  row_header_enum={}  col_header_enum={}  use_min_max=off  min_val=-inf  max_val=inf  use_precision=off  precision=''  gain=1  offset=0  exp=1  use_mototune_group=off  mototune_group=motohawk_vardec_path(gcb)
  motohawk_calibration2 : MotoHawk_lib/Calibration & Probing Blocks/motohawk_calibration  nam='Vehicle_Speed_Sensor_Circuit_Low_Fault'  val=300  storage=Calibration  show_more=off  name_source=Use Parameter  data_type=Inherit from 'Default Value'  read_level=1  write_level=1  ovr_cals=on  view_as=Number  enum_struct={'Disabled', 'Enabled'}  vector_style=Wide Row  use_help_units=off  help=''  units=''  use_header_enum=off  row_header_enum={}  col_header_enum={}  use_min_max=off  min_val=-inf  max_val=inf  use_precision=off  precision=''  gain=1  offset=0  exp=1  use_mototune_group=off  mototune_group=motohawk_vardec_path(gcb)
  motohawk_calibration3 : MotoHawk_lib/Calibration & Probing Blocks/motohawk_calibration  nam='Motor_Speed_TorqueRPM_Fault'  val=10  storage=Calibration  show_more=off  name_source=Use Parameter  data_type=Inherit from 'Default Value'  read_level=1  write_level=1  ovr_cals=on  view_as=Number  enum_struct={'Disabled', 'Enabled'}  vector_style=Wide Row  use_help_units=off  help=''  units=''  use_header_enum=off  row_header_enum={}  col_header_enum={}  use_min_max=off  min_val=-inf  max_val=inf  use_precision=off  precision=''  gain=1  offset=0  exp=1  use_mototune_group=off  mototune_group=motohawk_vardec_path(gcb)
  motohawk_calibration4 : MotoHawk_lib/Calibration & Probing Blocks/motohawk_calibration  nam='Motor_Speed_Torque_Fault'  val=100  storage=Calibration  show_more=off  name_source=Use Parameter  data_type=Inherit from 'Default Value'  read_level=1  write_level=1  ovr_cals=on  view_as=Number  enum_struct={'Disabled', 'Enabled'}  vector_style=Wide Row  use_help_units=off  help=''  units=''  use_header_enum=off  row_header_enum={}  col_header_enum={}  use_min_max=off  min_val=-inf  max_val=inf  use_precision=off  precision=''  gain=1  offset=0  exp=1  use_mototune_group=off  mototune_group=motohawk_vardec_path(gcb)
  motohawk_calibration7 : MotoHawk_lib/Calibration & Probing Blocks/motohawk_calibration  nam='Motor_Speed_Low_Fault'  val=-4000  storage=Calibration  show_more=off  name_source=Use Parameter  data_type=Inherit from 'Default Value'  read_level=1  write_level=1  ovr_cals=on  view_as=Number  enum_struct={'Disabled', 'Enabled'}  vector_style=Wide Row  use_help_units=off  help=''  units=''  use_header_enum=off  row_header_enum={}  col_header_enum={}  use_min_max=off  min_val=-inf  max_val=inf  use_precision=off  precision=''  gain=1  offset=0  exp=1  use_mototune_group=off  mototune_group=motohawk_vardec_path(gcb)
  motohawk_fault_def1 : MotoHawk_lib/Fault Management Blocks/motohawk_fault_def  nam='Vehicle_Speed_Sensor_Circuit_Low'  mode=Enabled  id=['P0502']  x=90  y=100  input_suspected=on  indeterminate=off  increment_xy=on  downsample_count=1  ovr_cals=on  ovr_actions=on  show_actions=on  action1_name='Wrench_Light'  action1_cond=Active  action2_name=''  action2_cond=(None)  action3_name=''  action3_cond=(None)  action4_name=''  action4_cond=(None)
  motohawk_fault_def2 : MotoHawk_lib/Fault Management Blocks/motohawk_fault_def  nam='Vehicle_Speed_Sensor_Erratic'  mode=Enabled  id=['P0503']  x=9  y=10  input_suspected=on  indeterminate=off  increment_xy=on  downsample_count=1  ovr_cals=on  ovr_actions=on  show_actions=on  action1_name='Wrench_Light'  action1_cond=Active  action2_name=''  action2_cond=(None)  action3_name=''  action3_cond=(None)  action4_name=''  action4_cond=(None)
  motohawk_fault_def3 : MotoHawk_lib/Fault Management Blocks/motohawk_fault_def  nam='Vehcile_Speed_Sensor_Malfunction'  mode=Enabled  id=['P0500']  x=9  y=10  input_suspected=on  indeterminate=off  increment_xy=on  downsample_count=1  ovr_cals=on  ovr_actions=on  show_actions=on  action1_name=''  action1_cond=(None)  action2_name=''  action2_cond=(None)  action3_name=''  action3_cond=(None)  action4_name=''  action4_cond=(None)
  motohawk_fault_def8 : MotoHawk_lib/Fault Management Blocks/motohawk_fault_def  nam='Vehicle_Speed_Sensor_Rang_Performance'  mode=Enabled  id=['P0501']  x=150  y=200  input_suspected=on  indeterminate=off  increment_xy=on  downsample_count=1  ovr_cals=on  ovr_actions=on  show_actions=on  action1_name='Wrench_Light'  action1_cond=Active  action2_name=''  action2_cond=(None)  action3_name=''  action3_cond=(None)  action4_name=''  action4_cond=(None)
  motohawk_fault_status : MotoHawk_lib/Fault Management Blocks/motohawk_fault_status  source=Lookup By Name  nam='Vehicle_Speed_Sensor_Rang_Performance'  status=Active
  motohawk_fault_status1 : MotoHawk_lib/Fault Management Blocks/motohawk_fault_status  source=Lookup By Name  nam='Vehicle_Speed_Sensor_Circuit_Low'  status=Active
  motohawk_fault_status2 : MotoHawk_lib/Fault Management Blocks/motohawk_fault_status  source=Lookup By Name  nam='Vehicle_Speed_Sensor_Erratic'  status=Active
  wires:
  In1/1 -> Bus Selector4/1, Bus Selector1/1, Bus Selector2/1
  Bus Selector4/1 -> Relational Operator7/1, Relational Operator1/1  "<IPT_MotorSpeed>"
  motohawk_calibration7/1 -> Relational Operator7/2
  motohawk_calibration1/1 -> Relational Operator1/2
  Relational Operator7/1 -> Logical Operator/1
  Relational Operator1/1 -> Logical Operator/2
  Logical Operator/1 -> motohawk_fault_def8/1
  Bus Selector1/1 -> Data Correction/1(torqueIn)  "<IPT_WheelTorqueDelivered>"
  Data Correction/1(torqueOut) -> Relational Operator2/1
  motohawk_calibration2/1 -> Relational Operator2/2
  Relational Operator2/1 -> Logical Operator1/1
  Bus Selector1/2 -> Relational Operator3/1  "<IPT_MotorSpeed>"
  motohawk_calibration3/1 -> Relational Operator3/2
  Relational Operator3/1 -> Logical Operator1/2
  Logical Operator1/1 -> motohawk_fault_def1/1
  Bus Selector2/1 -> Add/1, Unit Delay/1  "<IPT_MotorSpeed>"
  Unit Delay/1 -> Add/2
  Add/1 -> Abs/1
  Abs/1 -> Relational Operator/1
  motohawk_calibration4/1 -> Relational Operator/2
  Relational Operator/1 -> motohawk_fault_def2/1
  motohawk_fault_status1/1 -> Logical Operator2/2
  motohawk_fault_status2/1 -> Logical Operator2/3
  motohawk_fault_status/1 -> Logical Operator2/1
  Logical Operator2/1 -> motohawk_fault_def3/1

== system Mooventure2016_Rev5/Foreground/Control/Hybrid Control Code/CrawlHomeMode/SOC_RampOut ==
  note: 25 -- 100%
      | 20 -- 50%
      | 15 -- 0%
  Torque_In : Inport
  SOC : Inport  Port=2
  SoCBounds : Inport  Port=3
  Add : Sum  Inputs=+-
  Bus Selector : BusSelector  OutputSignals=CrawlHomeBoundSoC,SafetyModeBoundSoC
  Divide : Product  Inputs=*/
  Product : Product  RndMeth=Zero
  Saturation : Saturate  UpperLimit=1  LowerLimit=0
  Sum : Sum  Inputs=+-+
  Torque_Out : Outport
  wires:
  SOC/1 -> Sum/1
  Add/1 -> Sum/3, Divide/2
  Sum/1 -> Divide/1
  Divide/1 -> Saturation/1
  Torque_In/1 -> Product/1
  Product/1 -> Torque_Out/1
  Saturation/1 -> Product/2
  SoCBounds/1 -> Bus Selector/1
  Bus Selector/1 -> Add/1, Sum/2  "<CrawlHomeBoundSoC>"
  Bus Selector/2 -> Add/2  "<SafetyModeBoundSoC>"

== system Mooventure2016_Rev5/Foreground/Control/Hybrid Control Code/Cruise Control/Brake Disable ==
  Enable : EnablePort
  Constant : Constant  Value=0  OutDataTypeStr=boolean
  motohawk_data_write1 : MotoHawk_lib/Data Storage Blocks/motohawk_data_write  source=Lookup By Name  structure=Scalar  operation=Write entire data structure at once  sz_vec=9  sz_row=2  sz_col=9  typ=boolean  nam='CruiseOn'  checkNull=on  write_read_only=off  struct_inst_name=''  struct_name='MyStruct'
  wires:
  Constant/1 -> motohawk_data_write1/1

== system Mooventure2016_Rev5/Foreground/Control/Hybrid Control Code/Cruise Control/Speed Changing ==
  Set- : Inport
  Set+ : Inport  Port=2
  Detect Increase : simulink/Logic and Bit Operations/Detect Increase  SystemSampleTime=-1  vinit=0.0
  Detect Increase1 : simulink/Logic and Bit Operations/Detect Increase  SystemSampleTime=-1  vinit=0.0
  Logical Operator : Logic  AllPortsSameDT=off  OutDataTypeStr=boolean
  Logical Operator1 : Logic  AllPortsSameDT=off  OutDataTypeStr=boolean
  Speed Decrease : Subsystem  TreatAsAtomicUnit=on
  Speed Increase : Subsystem  TreatAsAtomicUnit=on
  motohawk_data_read : MotoHawk_lib/Data Storage Blocks/motohawk_data_read  source=Lookup By Name  structure=Scalar  operation=Read scalar from location by index  sz_vec=4  sz_row=2  sz_col=3  typ=boolean  nam='CruiseOn'  checkNull=on  struct_inst_name='MyData'  struct_nam='MyStruct'
  wires:
  motohawk_data_read/1 -> Logical Operator/1, Logical Operator1/1
  Set-/1 -> Detect Increase/1
  Detect Increase/1 -> Logical Operator/2
  Set+/1 -> Detect Increase1/1
  Detect Increase1/1 -> Logical Operator1/2
  Logical Operator/1 -> Speed Decrease/Enable
  Logical Operator1/1 -> Speed Increase/Enable

== system Mooventure2016_Rev5/Foreground/Control/Hybrid Control Code/Cruise Control/Speed Control ==
  Torque : Inport
  CurrentSpeed : Inport  Port=2
  DesiredSpeed : Inport  Port=3
  SystemEnable : Inport  Port=4
  Detect Rise Positive : simulink/Logic and Bit Operations/Detect Rise Positive  SystemSampleTime=-1  vinit=0
  PID With Damper Terms (Tunable) : Subsystem  AncestorBlock=motohawk_control_primitives_lib/PID With Damper Terms (Tunable)  mask(PID with Damper Terms (Tunable)){nam='Electronic Throttle Control', prefix='ETC_', samp_time=-1, units='', grp=motohawk_vardec_path(gcb)}
      mask prompts: nam "Name"; samp_time "Sample Time"; grp "MotoTune Group String"
      mask help:
      | This block wraps a 'PID With Damper Terms' block to provide calibrations and probes for most parameters.
      |
      | If 'Sample Time' is -1, then extra code and RAM will be generated to dynamically calculate dt.
      mask Display:
      | patch([0 0 1 1], [0 0.075 0.075 0], [230/255 0/255 0/255])
      | patch([0 0 1 1], [0.025 0.05 0.05 0.025], [150/255 0/255 0/255])
      | patch([0 0 1 1], [0 0.025 0.025 0], [0/255 0/255 0/255])
      | 
      | disp([nam '\n(PIDD)']);
  Switch : Switch  Threshold=1
  motohawk_data_read1 : MotoHawk_lib/Data Storage Blocks/motohawk_data_read  source=Lookup By Name  structure=Scalar  operation=Read scalar from location by index  sz_vec=4  sz_row=2  sz_col=3  typ=boolean  nam='CruiseOn'  checkNull=on  struct_inst_name='MyData'  struct_nam='MyStruct'
  motohawk_interpolation_1d : MotoHawk_lib/Lookup Tables/motohawk_interpolation_1d  nam='Cruise_Control_Map'  table_data=[0:15:1800]  show_more=on  data_type=double  storage=NonAdaptive  read_level=1  write_level=1  ovr_cals=on  use_help=off  help=''  units=''  use_min_max=off  min_val=0  max_val=1  use_precision=off  precision='1.2'  gain=1  offset=0  exp=1  use_links=on  prelookup_block='Cruise_Control_Pre'  output_name=''  use_mototune_group=off  mototune_group=motohawk_vardec_path(gcb)
  motohawk_prelookup : MotoHawk_lib/Lookup Tables/motohawk_prelookup  nam='Cruise_Control_Pre'  breakpoint_data=[0:1:120]  show_more=on  data_type=double  storage=Constant  read_level=1  write_level=1  ovr_cals=on  use_help=off  help=''  units=''  use_min_max=off  min_val=-inf  max_val=inf  use_precision=off  precision=''  gain=1  offset=0  exp=1  use_links=off  input_name=''  use_mototune_group=off  mototune_group=motohawk_vardec_path(gcb)
  TorqueOut : Outport
  wires:
  SystemEnable/1 -> Switch/2
  Torque/1 -> Switch/3
  Switch/1 -> TorqueOut/1
  CurrentSpeed/1 -> PID With Damper Terms (Tunable)/1(Actual)
  DesiredSpeed/1 -> PID With Damper Terms (Tunable)/2(SetPoint)
  Detect Rise Positive/1 -> PID With Damper Terms (Tunable)/3(ResetITerm)
  motohawk_data_read1/1 -> Detect Rise Positive/1
  motohawk_prelookup/1 -> motohawk_interpolation_1d/1
  PID With Damper Terms (Tunable)/1(Out) -> motohawk_prelookup/1
  motohawk_interpolation_1d/1 -> Switch/1
